simulink model "task3_2"  (R2024a)
settings: Solver=VariableStepAuto  StartTime=0.0  StopTime=100  RelTol=1e-3
undefined symbols (not defined in the file): B_eta, L, ss_gen_disc, ss_plant_discrete, T
settings Model: Creator=vladislav  LastModifiedBy=vladislav

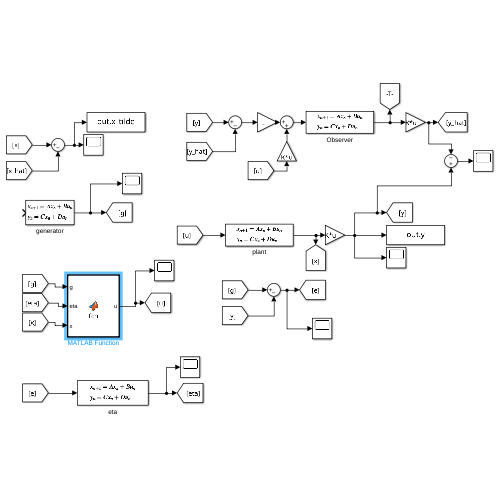
[thumbnail: Simulink's stored preview of the top-level diagram]
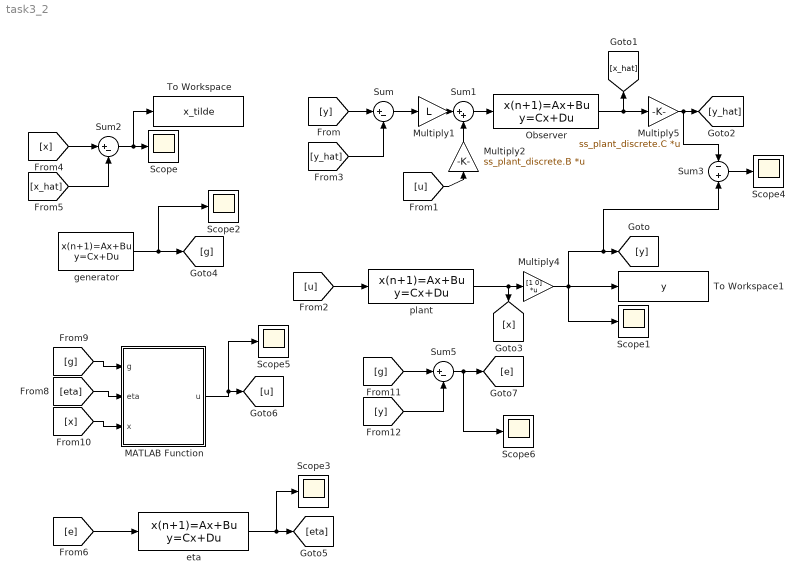
== system task3_2 ==
  MATLAB Function : MATLAB Function  TreatAsAtomicUnit=on
  Multiply1 : Gain  Gain=L
  Multiply2 : Gain  Gain=ss_plant_discrete.B  Multiplication=Matrix(K*u)
  Multiply4 : Gain  Gain=[1 0]  Multiplication=Matrix(K*u)
  Multiply5 : Gain  Gain=ss_plant_discrete.C  Multiplication=Matrix(K*u)
  Observer : DiscreteStateSpace  A=ss_plant_discrete.A  B=[1 0; 0 1]  C=eye(2)  D=[0 0; 0 0]  InitialCondition=[3 2]  SampleTime=T
  Scope{,1..6} (7 alike) : Scope
  Sum : Sum  Inputs=|+-
  Sum1 : Sum  Inputs=|++
  Sum2 : Sum  Inputs=|+-
  Sum3 : Sum  Inputs=-+
  Sum5 : Sum  Inputs=|+-
  To Workspace : ToWorkspace  VariableName=x_tilde  SaveFormat=Timeseries  SampleTime=-1
  To Workspace1 : ToWorkspace  VariableName=y  SaveFormat=Timeseries  SampleTime=-1
  eta : DiscreteStateSpace  A=ss_gen_disc.A  B=B_eta  C=[1 0; 0 1]  D=[0; 0]  InitialCondition=[0 1]  SampleTime=T
  generator : DiscreteStateSpace  A=ss_gen_disc.A  B=ss_gen_disc.B  C=ss_gen_disc.C  D=ss_gen_disc.D  InitialCondition=[0 1]  SampleTime=T
  plant : DiscreteStateSpace  A=ss_plant_discrete.A  B=ss_plant_discrete.B  C=[1 0; 0 1]  D=[0; 0]  InitialCondition=[1 1]  SampleTime=T
  wires:
  plant/1 -> [x], Multiply4/1
  [y] -> Sum/1
  Sum/1 -> Multiply1/1
  Multiply1/1 -> Sum1/1
  Sum1/1 -> Observer/1
  Observer/1 -> Multiply5/1, [x_hat]
  Multiply2/1 -> Sum1/2
  [u] -> plant/1
  [y_hat] -> Sum/2
  Multiply4/1 -> Sum3/2, [y], To Workspace1/1, Scope1/1
  [x] -> Sum2/1
  [x_hat] -> Sum2/2
  Sum2/1 -> To Workspace/1, Scope/1
  generator/1 -> Scope2/1, [g]
  [u] -> Multiply2/1
  Multiply5/1 -> Sum3/1, [y_hat]
  [e] -> eta/1
  eta/1 -> Scope3/1, [eta]
  [eta] -> MATLAB Function/2(eta)
  [g] -> MATLAB Function/1(g)
  [x] -> MATLAB Function/3(x)
  MATLAB Function/1(u) -> Scope5/1, [u]
  Sum5/1 -> Scope6/1, [e]
  [y] -> Sum5/2
  [g] -> Sum5/1
  Sum3/1 -> Scope4/1

== matlab function task3_2/MATLAB Function ==
  data: g input; u output; eta input; x input; K_bar parameter
function u = fcn(g, eta, x, K_bar)

u = -K_bar(1:2) * eta;
u = u - K_bar(3:4) * x;
u = u + g * K_bar(1)
